simulink model "drone_estimator_angle_dynamics"  (R2024a)
settings: Solver=FixedStepAuto  StartTime=0.0  StopTime=30  FixedStep=0.001  RelTol=1e-3
InitFcn:
  | os = 0.15;
  | zeta = -log(os)/sqrt(pi^2+(log(os))^2);
  | ts = 0.2;
  | wn = 4/zeta/ts;
  | kx = wn^2 - 1;
  | kf = 2 * zeta * wn;
  | Kx = eye(2) * kx;
  | Kf = eye(2) * kf;
  | 
  | 
  | os_des = 0.1;
  | zeta_des = -log(os_des)/sqrt(pi^2+(log(os_des))^2);
  | ts_des = 1;
  | wn_des = 4/zeta_des/ts_des;
  | b_des = wn_des^2;
  | a_des = 2 * zeta_des * wn_des;
undefined symbols (not defined in the file or in its folder): e0_0, e1_0, e2_0, e3_0, q0, QP, vec
libraries: sharedtransform x12, dspsigops x12, sharedutil x6, simulink x3
(part 2 of 2)

== system drone_estimator_angle_dynamics/Quaternion Command/Filtering Command Signal ==
  Command : Inport
  In Bus Element : Inport  Port=2  PortName=States  Element=Euler.ϕ
  In Bus Element2 : Inport  Port=2  PortName=States  Element=Euler.θ
  In Bus Element1 : Inport  Port=2  PortName=States  Element=Euler.Ψ
  Demux : Demux  Outputs=3
  Mux : Mux  Inputs=3
  Pitch Dynamic Sat : Subsystem  mask{Range=PitchRange}
      mask prompts: Range "Saturation Range"
      mask TypeOptions Range: range/Value
  Pitch Rate Limiter : RateLimiter  RisingSlewLimit=PitchRisingSlewLimit  FallingSlewLimit=PitchFallingSlewLimit  SampleTimeMode=inherited
  Roll Dynamic Sat : Subsystem  mask{Range=RollRange}
      mask prompts: Range "Saturation Range"
      mask TypeOptions Range: range/Value
  Roll Rate Limiter : RateLimiter  RisingSlewLimit=RollRisingSlewLimit  FallingSlewLimit=RollFallingSlewLimit  SampleTimeMode=inherited
  Yaw Dynamic Sat : Subsystem  mask{Range=YawRange}
      mask prompts: Range "Saturation Range"
      mask TypeOptions Range: range/Value
  Yaw Rate Limiter : RateLimiter  RisingSlewLimit=YawRisingSlewLimit  FallingSlewLimit=YawFallingSlewLimit  SampleTimeMode=inherited
  Filtered : Outport
  wires:
  Yaw Dynamic Sat/1(Saturated Command) -> Yaw Rate Limiter/1
  Mux/1 -> Filtered/1
  Pitch Dynamic Sat/1(Saturated Command) -> Pitch Rate Limiter/1
  Demux/3 -> Yaw Dynamic Sat/2(Command)
  Demux/1 -> Roll Dynamic Sat/2(Command)
  In Bus Element/1 -> Roll Dynamic Sat/1(State)
  Roll Dynamic Sat/1(Saturated Command) -> Roll Rate Limiter/1
  Demux/2 -> Pitch Dynamic Sat/2(Command)
  Command/1 -> Demux/1
  In Bus Element1/1 -> Yaw Dynamic Sat/1(State)
  In Bus Element2/1 -> Pitch Dynamic Sat/1(State)
  Roll Rate Limiter/1 -> Mux/1
  Pitch Rate Limiter/1 -> Mux/2
  Yaw Rate Limiter/1 -> Mux/3

== system drone_estimator_angle_dynamics/Quaternion Command/Rotation Interpolation ==
  DCM : Inport
  In Bus Element1 : Inport  Port=2  PortName=States  Element=Quat
  In Bus Element : Inport  Port=2  PortName=States  Element=Euler
  Quaternion Interpolation : QuatInterp
  Quaternions to Direction Cosine Matrix1 : sharedtransform/Quaternions to  Direction Cosine Matrix  aMode=aMode
      settings: LibrarySourceBlock=|
      | aerolibtransform2/Quaternions to
      | Direction Cosine Matrix
  Subsystem : Subsystem
  Sum1 : Sum  Inputs=|+-
  alpha : Subsystem
  Rot : Outport
  wires:
  Subsystem/2(angles) -> Sum1/1
  Quaternion Interpolation/1 -> Quaternions to Direction Cosine Matrix1/1
  Quaternions to Direction Cosine Matrix1/1 -> Rot/1
  alpha/1(alpha) -> Quaternion Interpolation/3
  In Bus Element1/1 -> Quaternion Interpolation/1
  Subsystem/1(Quaternion) -> Quaternion Interpolation/2
  Sum1/1 -> alpha/1(angle difference)
  DCM/1 -> Subsystem/1(DCM)
  In Bus Element/1 -> Sum1/2

== system drone_estimator_angle_dynamics/Quaternion Command/ToGo ==
  DCM : Inport
  Bus Creator3 : BusCreator  Inputs=3
  Demux3 : Demux  Outputs=3
  Direction Cosine Matrix to Rotation Angles : sharedtransform/Direction Cosine Matrix to Rotation Angles  rotationOrder=ZYX  aMode=aMode  action=None  tolerance=eps(2)
      settings: LibrarySourceBlock=|
      | aerolibtransform2/Direction Cosine Matrix
      | to Rotation Angles
  Selector1 : Selector  InputPortWidth=3  IndexOptions=Index vector (dialog)  Indices=[3 2 1]  OutputSizes=1
  Unwrap2 : dspsigops/Unwrap  tol=2*pi  InputProcessing=Columns as channels (frame based)  running=off
  Unwrap3 : dspsigops/Unwrap  tol=2*pi  InputProcessing=Columns as channels (frame based)  running=off
  Unwrap4 : dspsigops/Unwrap  tol=2*pi  InputProcessing=Columns as channels (frame based)  running=off
  tag scope: Euler_c=global
  wires:
  Unwrap3/1 -> Bus Creator3/1  "ϕc"
  Demux3/1 -> Unwrap3/1
  Unwrap2/1 -> Bus Creator3/2  "θc"
  Demux3/3 -> Unwrap4/1  "Ψc"
  Bus Creator3/1 -> [Euler_c]
  Direction Cosine Matrix to Rotation Angles/1 -> Selector1/1
  Demux3/2 -> Unwrap2/1
  DCM/1 -> Demux3/1
  Unwrap4/1 -> Bus Creator3/3  "Ψc"

== system drone_estimator_angle_dynamics/Quaternion Command/quaternion ==
  angle : Inport
  vec : Inport  Port=2
  Gain : Gain  Gain=1/2
  Mux : Mux  Inputs=2
  Product : Product
  Quaternion Normalize : sharedutil/Quaternion Normalize  aMode=aMode
  Quaternions to Direction Cosine Matrix : sharedtransform/Quaternions to  Direction Cosine Matrix  aMode=aMode
      settings: LibrarySourceBlock=|
      | aerolibtransform2/Quaternions to
      | Direction Cosine Matrix
  Rate Limiter : RateLimiter  RisingSlewLimit=0.4  FallingSlewLimit=-0.4  SampleTimeMode=inherited
  Trigonometric Function : Trigonometry
  Trigonometric Function1 : Trigonometry  Operator=cos
  rot : Outport
  wires:
  Trigonometric Function1/1 -> Mux/1
  Mux/1 -> Quaternion Normalize/1
  Product/1 -> Mux/2
  Trigonometric Function/1 -> Product/1
  Gain/1 -> Trigonometric Function1/1, Trigonometric Function/1
  Rate Limiter/1 -> Product/2
  angle/1 -> Gain/1
  Quaternion Normalize/1 -> Quaternions to Direction Cosine Matrix/1
  vec/1 -> Rate Limiter/1
  Quaternions to Direction Cosine Matrix/1 -> rot/1

== system drone_estimator_angle_dynamics/Quaternion Command/to Rotation Mat ==
  Euler : Inport
  Rotation Angles to Direction Cosine Matrix : sharedtransform/Rotation Angles to Direction Cosine Matrix  rotationOrder=ZYX  aMode=aMode
  Selector : Selector  InputPortWidth=3  IndexOptions=Index vector (dialog)  Indices=[3 2 1]  OutputSizes=1
  rot : Outport
  wires:
  Selector/1 -> Rotation Angles to Direction Cosine Matrix/1
  Rotation Angles to Direction Cosine Matrix/1 -> rot/1
  Euler/1 -> Selector/1

== system drone_estimator_angle_dynamics/Rotational Matrix Controller/Quaternion Dynamics ==
  R : Inport
  Add2 : Sum  Inputs=|+-
  "Desired Rotaion Dynamic Gain " : Gain  Gain=DesiredRotaionDynamciGain
  Euler Command : Subsystem
  Euler Desired : Subsystem
  Quaternion Command : Subsystem
  Rotaion Integration : Integrator  InitialCondition=InitialCondition  ContinuousStateAttributes='qd'
  Scope : Scope
  Rd : Outport
  Rd_dot : Outport  Port=2
  wires:
  Rotaion Integration/1 -> Euler Desired/1(DCM), Add2/2, Rd/1, Scope/1
  Add2/1 -> Rd_dot/1, "Desired Rotaion Dynamic Gain "/1
  "Desired Rotaion Dynamic Gain "/1 -> Rotaion Integration/1
  R/1 -> Quaternion Command/1(DCM), Euler Command/1(DCM), Add2/1

== system drone_estimator_angle_dynamics/Rotational Matrix Controller/Rotational Controller ==
  Rd : Inport
  Rd_dot : Inport  Port=2
  Rot : Inport  Port=3
  Kr : Constant  Value=RotationControlGain
  MATLAB Function : MATLAB Function  TreatAsAtomicUnit=on
  MATLAB Function1 : MATLAB Function  TreatAsAtomicUnit=on
  Manual Switch : ManualSwitch  CurrentSetting=0
  Manual Switch2 : ManualSwitch  CurrentSetting=0
  "Rd " : InportShadow
  "Rd_dot " : InportShadow  Port=2
  "Rot " : InportShadow  Port=3
  Scope : Scope
  Scope1 : Scope
  wc : Outport
  tag scope: sr=global
  wires:
  Rd/1 -> MATLAB Function/3(Rd)
  MATLAB Function/1(sr) -> Manual Switch2/1
  Kr/1 -> MATLAB Function1/1(Kr), MATLAB Function/1(Kr)
  MATLAB Function/2(wc) -> Manual Switch/1
  Rd_dot/1 -> MATLAB Function/4(Rd_dot)
  Manual Switch/1 -> wc/1
  "Rd_dot "/1 -> MATLAB Function1/4(Rd_dot)
  "Rd "/1 -> MATLAB Function1/3(Rd)
  MATLAB Function1/2(wc) -> Manual Switch/2
  MATLAB Function/3(Re) -> Scope/1
  Manual Switch2/1 -> [sr]
  MATLAB Function1/1(sr) -> Manual Switch2/2
  MATLAB Function1/3(Re) -> Scope1/1
  "Rot "/1 -> MATLAB Function1/2(R)
  Rot/1 -> MATLAB Function/2(R)

== system drone_estimator_angle_dynamics/Angular Rate Controller/Dynamic Surface Angular Rate Controller/Angular Rate Desired Dynamics ==
  wc : Inport
  Desired Angular Rate Integaration : Integrator  InitialCondition=DesiredAngularRateInitCond
  Sum : Sum  Inputs=|+-
  tau : Gain  Gain=OmegaTimeConstant
  wd : Outport
  wd dot : Outport  Port=2
  wires:
  Sum/1 -> tau/1
  Desired Angular Rate Integaration/1 -> wd/1, Sum/2
  wc/1 -> Sum/1
  tau/1 -> wd dot/1, Desired Angular Rate Integaration/1

== system drone_estimator_angle_dynamics/Estimator/Model Predictor/Nonlinear function estimator ==
  e : Inport
  Add1 : Sum
  Gain : Gain  Gain=5
  Gain1 : Gain  Gain=2
  Integrator : Integrator
  fest : Outport
  tag scope: Fest=global
  wires:
  e/1 -> Gain1/1, Integrator/1
  Gain1/1 -> Add1/1
  Add1/1 -> fest/1, [Fest]
  Gain/1 -> Add1/2
  Integrator/1 -> Gain/1

== system drone_estimator_angle_dynamics/Estimator/Model Predictor/Subsystem1 ==
  xe : Inport
  x : Inport  Port=2
  Bus Creator1 : BusCreator  Inputs=3
  Bus Selector : BusSelector  OutputSignals=w.p,w.q,w.r  OutputAsBus=on
  Bus Selector1 : BusSelector  OutputSignals=p,q,r  OutputAsBus=on
  Demux : Demux  Outputs=3
  Reshape1 : Reshape  OutputDimensionality=Column vector (2-D)
  Reshape4 : Reshape  OutputDimensionality=Column vector (2-D)
  Subtract : Sum  Inputs=+-
  er : Outport
  tag scope: we_est=global
  wires:
  Demux/3 -> Bus Creator1/3  "er"
  Reshape4/1 -> Subtract/1
  Bus Selector1/1 -> Reshape1/1
  Reshape1/1 -> Subtract/2
  Demux/2 -> Bus Creator1/2  "eq"
  x/1 -> Bus Selector/1
  Bus Creator1/1 -> [we_est]
  Demux/1 -> Bus Creator1/1  "ep"
  Bus Selector/1 -> Reshape4/1
  xe/1 -> Bus Selector1/1
  Subtract/1 -> Demux/1, er/1

== system drone_estimator_angle_dynamics/Estimator/Model Predictor1/Centrifugal Moments ==
  ω : Inport
  Inertia : Inport  Port=2
  3x3 Cross Product : sharedutil/3x3 Cross Product  aMode=aMode
  Product : Product  Multiplication=Matrix(*)  InputSameDT=on  SaturateOnIntegerOverflow=on  OutDataTypeStr=Inherit: Same as first input
  To1D : Reshape
  ToVec : Reshape  OutputDimensionality=Column vector (2-D)
  (I * ω) x ω : Outport
  wires:
  Inertia/1 -> Product/1
  To1D/1 -> 3x3 Cross Product/1  "I * ω"
  3x3 Cross Product/1 -> (I * ω) x ω/1
  ω/1 -> ToVec/1, 3x3 Cross Product/2
  Product/1 -> To1D/1
  ToVec/1 -> Product/2

== system drone_estimator_angle_dynamics/Estimator/Model Predictor1/Subsystem ==
  (I * ω) x ω : Inport
  e : Inport  Port=2
  Add1 : Sum  Inputs=+++
  Gain : Gain  Gain=5
  Gain1 : Gain  Gain=2
  Integrator : Integrator
  fest : Outport
  tag scope: Fest=global
  wires:
  (I * ω) x ω/1 -> Add1/3
  Integrator/1 -> Gain/1
  Gain/1 -> Add1/2
  Add1/1 -> [Fest], fest/1
  Gain1/1 -> Add1/1
  e/1 -> Integrator/1, Gain1/1

== system drone_estimator_angle_dynamics/Estimator/Model Predictor1/Subsystem1 ==
  xe : Inport
  x : Inport  Port=2
  Bus Creator1 : BusCreator  Inputs=3
  Bus Selector : BusSelector  OutputSignals=w.p,w.q,w.r  OutputAsBus=on
  Bus Selector1 : BusSelector  OutputSignals=p,q,r  OutputAsBus=on
  Demux : Demux  Outputs=3
  Reshape1 : Reshape  OutputDimensionality=Column vector (2-D)
  Reshape4 : Reshape  OutputDimensionality=Column vector (2-D)
  Subtract : Sum  Inputs=+-
  er : Outport
  tag scope: we_est=global
  wires:
  Subtract/1 -> Demux/1
  xe/1 -> Bus Selector1/1
  Bus Selector/1 -> Reshape4/1
  Demux/1 -> Bus Creator1/1  "ep"
  Bus Creator1/1 -> er/1, [we_est]
  x/1 -> Bus Selector/1
  Demux/2 -> Bus Creator1/2  "eq"
  Reshape1/1 -> Subtract/2
  Bus Selector1/1 -> Reshape1/1
  Reshape4/1 -> Subtract/1
  Demux/3 -> Bus Creator1/3  "er"

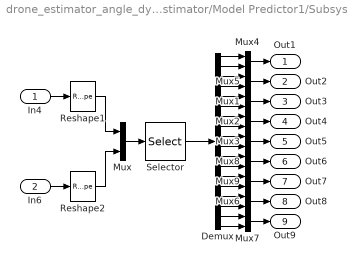
== system drone_estimator_angle_dynamics/Estimator/Model Predictor1/Subsystem2 ==
  In4 : Inport
  In6 : Inport  Port=2
  Demux : Demux  Outputs=18
  Mux{,1..9} (10 alike) : Mux  Inputs=2
  Reshape1 : Reshape
  Reshape2 : Reshape
  Selector : Selector  InputPortWidth=18  IndexOptions=Index vector (dialog)  Indices=[1 10 2 11 3 12 4 13 5 14 6 15 7 16 8 17 9 18]  OutputSizes=1
  Out1 : Outport
  Out2 : Outport  Port=2
  Out3 : Outport  Port=3
  Out4 : Outport  Port=4
  Out5 : Outport  Port=5
  Out6 : Outport  Port=6
  Out7 : Outport  Port=7
  Out8 : Outport  Port=8
  Out9 : Outport  Port=9
  wires:
  Demux/12 -> Mux8/2
  Demux/13 -> Mux9/1
  Demux/14 -> Mux9/2
  Demux/15 -> Mux6/1
  Demux/16 -> Mux6/2
  Demux/17 -> Mux7/1
  Demux/18 -> Mux7/2
  Demux/11 -> Mux8/1
  Demux/10 -> Mux3/2
  Demux/9 -> Mux3/1
  Demux/8 -> Mux2/2
  Demux/7 -> Mux2/1
  Demux/6 -> Mux1/2
  Demux/5 -> Mux1/1
  Demux/4 -> Mux5/2
  Demux/3 -> Mux5/1
  Demux/2 -> Mux4/2
  Demux/1 -> Mux4/1
  Selector/1 -> Demux/1
  Mux/1 -> Selector/1
  Mux8/1 -> Out6/1
  Mux9/1 -> Out7/1
  Mux7/1 -> Out9/1
  Mux6/1 -> Out8/1
  Mux3/1 -> Out5/1
  Mux1/1 -> Out3/1
  Mux2/1 -> Out4/1
  Mux5/1 -> Out2/1
  In6/1 -> Reshape2/1
  Reshape2/1 -> Mux/2
  In4/1 -> Reshape1/1
  Reshape1/1 -> Mux/1
  Mux4/1 -> Out1/1

== system drone_estimator_angle_dynamics/Estimator/Model Predictor1/Subsystem3 ==
  In1 : Inport
  In2 : Inport  Port=2
  Demux : Demux  Outputs=3
  Demux1 : Demux  Outputs=3
  Mux10 : Mux  Inputs=2
  Mux11 : Mux  Inputs=2
  Mux9 : Mux  Inputs=2
  Out1 : Outport
  Out2 : Outport  Port=2
  Out3 : Outport  Port=3
  wires:
  Demux/3 -> Mux11/1
  Mux9/1 -> Out1/1
  Demux1/1 -> Mux9/2
  Demux/2 -> Mux10/1
  Demux/1 -> Mux9/1
  Demux1/3 -> Mux11/2
  Demux1/2 -> Mux10/2
  Mux11/1 -> Out3/1
  Mux10/1 -> Out2/1
  In1/1 -> Demux/1
  In2/1 -> Demux1/1

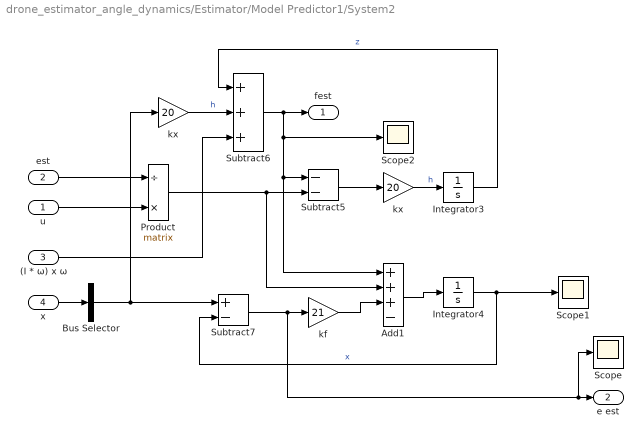
== system drone_estimator_angle_dynamics/Estimator/Model Predictor1/System2 ==
  u : Inport
  est : Inport  Port=2
  (I * ω) x ω : Inport  Port=3
  x : Inport  Port=4
  Add1 : Sum  Inputs=+++-
  Bus Selector : BusSelector  OutputSignals=w.p,w.q,w.r  OutputAsBus=on
  Integrator3 : Integrator  InitialCondition=zeros(3,1)
  Integrator4 : Integrator  InitialCondition=zeros(3,1)
  Product : Product  Inputs=/*  Multiplication=Matrix(*)
  Scope : Scope
  Scope1 : Scope
  Scope2 : Scope
  Subtract5 : Sum  Inputs=--
  Subtract6 : Sum  Inputs=+++
  Subtract7 : Sum  Inputs=+-
  kf : Gain  Gain=21
  kx : Gain  Gain=20
  "kx " : Gain  Gain=20
  fest : Outport
  e est : Outport  Port=2
  wires:
  (I * ω) x ω/1 -> Subtract6/3
  Bus Selector/1 -> kx/1, Subtract7/1
  u/1 -> Product/2
  est/1 -> Product/1
  Subtract7/1 -> kf/1, Scope/1, e est/1
  x/1 -> Bus Selector/1
  kf/1 -> Add1/3
  Integrator4/1 -> Subtract7/2, Scope1/1  "x"
  Add1/1 -> Integrator4/1
  Product/1 -> Subtract5/2, Add1/2
  Subtract6/1 -> fest/1, Subtract5/1, Add1/1, Scope2/1
  "kx "/1 -> Integrator3/1  "h"
  Subtract5/1 -> "kx "/1
  Integrator3/1 -> Subtract6/1  "z"
  kx/1 -> Subtract6/2  "h"

== system drone_estimator_angle_dynamics/Estimator1/Model Predictor/Nonlinear function estimator ==
  e : Inport
  Add1 : Sum
  Gain : Gain  Gain=5
  Gain1 : Gain  Gain=2
  Integrator : Integrator
  fest : Outport
  tag scope: Fest=global
  wires:
  Integrator/1 -> Gain/1
  Gain/1 -> Add1/2
  Add1/1 -> [Fest], fest/1
  Gain1/1 -> Add1/1
  e/1 -> Integrator/1, Gain1/1

== system drone_estimator_angle_dynamics/Estimator1/Model Predictor/Subsystem1 ==
  xe : Inport
  x : Inport  Port=2
  Bus Creator1 : BusCreator  Inputs=3
  Bus Selector : BusSelector  OutputSignals=w.p,w.q,w.r  OutputAsBus=on
  Bus Selector1 : BusSelector  OutputSignals=p,q,r  OutputAsBus=on
  Demux : Demux  Outputs=3
  Reshape1 : Reshape  OutputDimensionality=Column vector (2-D)
  Reshape4 : Reshape  OutputDimensionality=Column vector (2-D)
  Subtract : Sum  Inputs=+-
  er : Outport
  tag scope: we_est=global
  wires:
  Subtract/1 -> er/1, Demux/1
  xe/1 -> Bus Selector1/1
  Bus Selector/1 -> Reshape4/1
  Demux/1 -> Bus Creator1/1  "ep"
  Bus Creator1/1 -> [we_est]
  x/1 -> Bus Selector/1
  Demux/2 -> Bus Creator1/2  "eq"
  Reshape1/1 -> Subtract/2
  Bus Selector1/1 -> Reshape1/1
  Reshape4/1 -> Subtract/1
  Demux/3 -> Bus Creator1/3  "er"

== system drone_estimator_angle_dynamics/Estimator1/Model Predictor1/Centrifugal Moments ==
  ω : Inport
  Inertia : Inport  Port=2
  3x3 Cross Product : sharedutil/3x3 Cross Product  aMode=aMode
  Product : Product  Multiplication=Matrix(*)  InputSameDT=on  SaturateOnIntegerOverflow=on  OutDataTypeStr=Inherit: Same as first input
  To1D : Reshape
  ToVec : Reshape  OutputDimensionality=Column vector (2-D)
  (I * ω) x ω : Outport
  wires:
  ToVec/1 -> Product/2
  Product/1 -> To1D/1
  ω/1 -> 3x3 Cross Product/2, ToVec/1
  3x3 Cross Product/1 -> (I * ω) x ω/1
  To1D/1 -> 3x3 Cross Product/1  "I * ω"
  Inertia/1 -> Product/1

== system drone_estimator_angle_dynamics/Estimator1/Model Predictor1/Subsystem ==
  (I * ω) x ω : Inport
  e : Inport  Port=2
  Add1 : Sum  Inputs=+++
  Gain : Gain  Gain=5
  Gain1 : Gain  Gain=2
  Integrator : Integrator
  fest : Outport
  tag scope: Fest=global
  wires:
  e/1 -> Gain1/1, Integrator/1
  Gain1/1 -> Add1/1
  Add1/1 -> fest/1, [Fest]
  Gain/1 -> Add1/2
  Integrator/1 -> Gain/1
  (I * ω) x ω/1 -> Add1/3

== system drone_estimator_angle_dynamics/Estimator1/Model Predictor1/Subsystem1 ==
  xe : Inport
  x : Inport  Port=2
  Bus Creator1 : BusCreator  Inputs=3
  Bus Selector : BusSelector  OutputSignals=w.p,w.q,w.r  OutputAsBus=on
  Bus Selector1 : BusSelector  OutputSignals=p,q,r  OutputAsBus=on
  Demux : Demux  Outputs=3
  Reshape1 : Reshape  OutputDimensionality=Column vector (2-D)
  Reshape4 : Reshape  OutputDimensionality=Column vector (2-D)
  Subtract : Sum  Inputs=+-
  er : Outport
  tag scope: we_est=global
  wires:
  Demux/3 -> Bus Creator1/3  "er"
  Reshape4/1 -> Subtract/1
  Bus Selector1/1 -> Reshape1/1
  Reshape1/1 -> Subtract/2
  Demux/2 -> Bus Creator1/2  "eq"
  x/1 -> Bus Selector/1
  Bus Creator1/1 -> [we_est], er/1
  Demux/1 -> Bus Creator1/1  "ep"
  Bus Selector/1 -> Reshape4/1
  xe/1 -> Bus Selector1/1
  Subtract/1 -> Demux/1

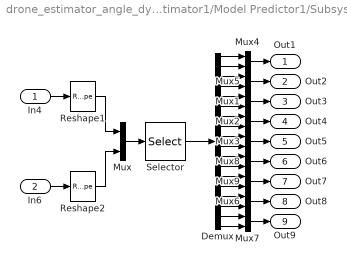
== system drone_estimator_angle_dynamics/Estimator1/Model Predictor1/Subsystem2 ==
  In4 : Inport
  In6 : Inport  Port=2
  Demux : Demux  Outputs=18
  Mux{,1..9} (10 alike) : Mux  Inputs=2
  Reshape1 : Reshape
  Reshape2 : Reshape
  Selector : Selector  InputPortWidth=18  IndexOptions=Index vector (dialog)  Indices=[1 10 2 11 3 12 4 13 5 14 6 15 7 16 8 17 9 18]  OutputSizes=1
  Out1 : Outport
  Out2 : Outport  Port=2
  Out3 : Outport  Port=3
  Out4 : Outport  Port=4
  Out5 : Outport  Port=5
  Out6 : Outport  Port=6
  Out7 : Outport  Port=7
  Out8 : Outport  Port=8
  Out9 : Outport  Port=9
  wires:
  Mux4/1 -> Out1/1
  Reshape1/1 -> Mux/1
  In4/1 -> Reshape1/1
  Reshape2/1 -> Mux/2
  In6/1 -> Reshape2/1
  Mux5/1 -> Out2/1
  Mux2/1 -> Out4/1
  Mux1/1 -> Out3/1
  Mux3/1 -> Out5/1
  Mux6/1 -> Out8/1
  Mux7/1 -> Out9/1
  Mux9/1 -> Out7/1
  Mux8/1 -> Out6/1
  Mux/1 -> Selector/1
  Selector/1 -> Demux/1
  Demux/1 -> Mux4/1
  Demux/2 -> Mux4/2
  Demux/3 -> Mux5/1
  Demux/4 -> Mux5/2
  Demux/5 -> Mux1/1
  Demux/6 -> Mux1/2
  Demux/7 -> Mux2/1
  Demux/8 -> Mux2/2
  Demux/9 -> Mux3/1
  Demux/10 -> Mux3/2
  Demux/11 -> Mux8/1
  Demux/18 -> Mux7/2
  Demux/17 -> Mux7/1
  Demux/16 -> Mux6/2
  Demux/15 -> Mux6/1
  Demux/14 -> Mux9/2
  Demux/13 -> Mux9/1
  Demux/12 -> Mux8/2

== system drone_estimator_angle_dynamics/Estimator1/Model Predictor1/Subsystem3 ==
  In1 : Inport
  In2 : Inport  Port=2
  Demux : Demux  Outputs=3
  Demux1 : Demux  Outputs=3
  Mux10 : Mux  Inputs=2
  Mux11 : Mux  Inputs=2
  Mux9 : Mux  Inputs=2
  Out1 : Outport
  Out2 : Outport  Port=2
  Out3 : Outport  Port=3
  wires:
  In2/1 -> Demux1/1
  In1/1 -> Demux/1
  Mux10/1 -> Out2/1
  Mux11/1 -> Out3/1
  Demux1/2 -> Mux10/2
  Demux1/3 -> Mux11/2
  Demux/1 -> Mux9/1
  Demux/2 -> Mux10/1
  Demux1/1 -> Mux9/2
  Mux9/1 -> Out1/1
  Demux/3 -> Mux11/1

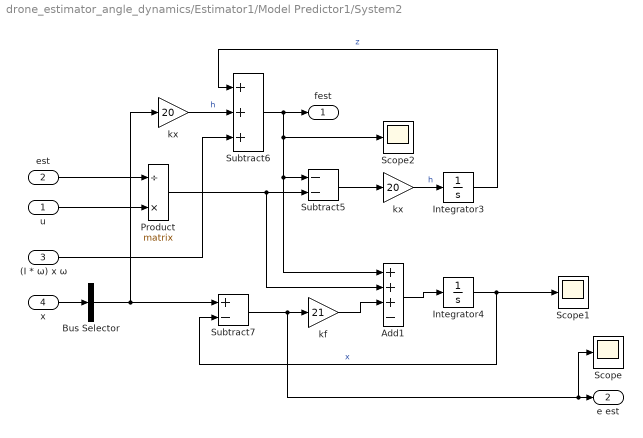
== system drone_estimator_angle_dynamics/Estimator1/Model Predictor1/System2 ==
  u : Inport
  est : Inport  Port=2
  (I * ω) x ω : Inport  Port=3
  x : Inport  Port=4
  Add1 : Sum  Inputs=+++-
  Bus Selector : BusSelector  OutputSignals=w.p,w.q,w.r  OutputAsBus=on
  Integrator3 : Integrator  InitialCondition=zeros(3,1)
  Integrator4 : Integrator  InitialCondition=zeros(3,1)
  Product : Product  Inputs=/*  Multiplication=Matrix(*)
  Scope : Scope
  Scope1 : Scope
  Scope2 : Scope
  Subtract5 : Sum  Inputs=--
  Subtract6 : Sum  Inputs=+++
  Subtract7 : Sum  Inputs=+-
  kf : Gain  Gain=21
  kx : Gain  Gain=20
  "kx " : Gain  Gain=20
  fest : Outport
  e est : Outport  Port=2
  wires:
  kx/1 -> Subtract6/2  "h"
  Integrator3/1 -> Subtract6/1  "z"
  Subtract5/1 -> "kx "/1
  "kx "/1 -> Integrator3/1  "h"
  Subtract6/1 -> Scope2/1, Add1/1, Subtract5/1, fest/1
  Product/1 -> Add1/2, Subtract5/2
  Add1/1 -> Integrator4/1
  Integrator4/1 -> Scope1/1, Subtract7/2  "x"
  kf/1 -> Add1/3
  x/1 -> Bus Selector/1
  Subtract7/1 -> e est/1, Scope/1, kf/1
  est/1 -> Product/1
  u/1 -> Product/2
  Bus Selector/1 -> Subtract7/1, kx/1
  (I * ω) x ω/1 -> Subtract6/3

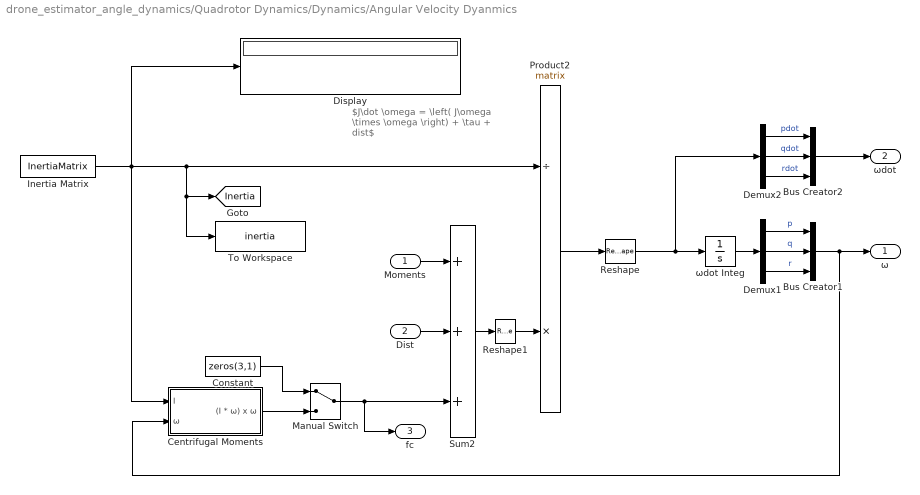
== system drone_estimator_angle_dynamics/Quadrotor Dynamics/Dynamics/Angular Velocity Dyanmics ==
  note: $J\dot \omega = \left( J\omega \times \omega \right) + \tau + dist$
  Moments : Inport  OutDataTypeStr=double
  Dist : Inport  Port=2  OutDataTypeStr=double
  Bus Creator1 : BusCreator  Inputs=3
  Bus Creator2 : BusCreator  Inputs=3
  Centrifugal Moments : Subsystem
  Constant : Constant  Value=zeros(3,1)
  Demux1 : Demux  Outputs=3
  Demux2 : Demux  Outputs=3
  Display : Display
  Inertia Matrix : Constant  Value=InertiaMatrix
  Manual Switch : ManualSwitch
  Product2 : Product  Inputs=/*  Multiplication=Matrix(*)  SaturateOnIntegerOverflow=on  OutDataTypeStr=Inherit: Same as first input
  Reshape : Reshape
  Reshape1 : Reshape  OutputDimensionality=Column vector (2-D)
  Sum2 : Sum  Inputs=+++  SaturateOnIntegerOverflow=on
  To Workspace : ToWorkspace  VariableName=inertia  SampleTime=-1
      settings: Save2DSignal=2-D array (concatenate along first dimension)
  ωdot Integ : Integrator  InitialCondition=OmegaInitialValues  ContinuousStateAttributes={'p', 'q', 'r'}
  ω : Outport
  ωdot : Outport  Port=2  OutDataTypeStr=double  Unit=rad/s^2  VectorParamsAs1DForOutWhenUnconnected=off
  fc : Outport  Port=3
  tag scope: Inertia=global
  wires:
  Product2/1 -> Reshape/1
  Reshape1/1 -> Product2/2
  Demux1/1 -> Bus Creator1/1  "p"
  ωdot Integ/1 -> Demux1/1
  Demux1/3 -> Bus Creator1/3  "r"
  Demux1/2 -> Bus Creator1/2  "q"
  Bus Creator1/1 -> ω/1, Centrifugal Moments/2(ω)
  Sum2/1 -> Reshape1/1
  Reshape/1 -> ωdot Integ/1, Demux2/1
  Demux2/2 -> Bus Creator2/2  "qdot"
  Demux2/3 -> Bus Creator2/3  "rdot"
  Demux2/1 -> Bus Creator2/1  "pdot"
  Bus Creator2/1 -> ωdot/1
  Inertia Matrix/1 -> To Workspace/1, [Inertia], Product2/1, Display/1, Centrifugal Moments/1(I)
  Moments/1 -> Sum2/1
  Manual Switch/1 -> fc/1, Sum2/3
  Centrifugal Moments/1((I * ω) x ω) -> Manual Switch/2
  Constant/1 -> Manual Switch/1
  Dist/1 -> Sum2/2

== system drone_estimator_angle_dynamics/Quadrotor Dynamics/Dynamics/Mixer ==
  Omegas : Inport
  Bus Creator : BusCreator  Inputs=4
  Constant : Constant  Value=ThustForceCoefficient
  Demux : Demux
  Matrix Multiply : Product  Multiplication=Matrix(*)
  Square : Math  Operator=square
  U : Outport
  wires:
  Bus Creator/1 -> U/1
  Demux/4 -> Bus Creator/4  "Tz"
  Demux/3 -> Bus Creator/3  "Ty"
  Demux/2 -> Bus Creator/2  "Tx"
  Demux/1 -> Bus Creator/1  "Th"
  Constant/1 -> Matrix Multiply/1
  Matrix Multiply/1 -> Demux/1
  Omegas/1 -> Matrix Multiply/2

== system drone_estimator_angle_dynamics/Quadrotor Dynamics/Dynamics/Quaternion Dynamics ==
  ω : Inport
  Quat to Euler : Subsystem
  Quaternion Dynamics : Subsystem
  Rotational Dynamics : Subsystem
  DCM_be : Outport  OutDataTypeStr=double  VectorParamsAs1DForOutWhenUnconnected=off
  Quat : Outport  Port=2  OutDataTypeStr=double  VectorParamsAs1DForOutWhenUnconnected=off
  Euler : Outport  Port=3  OutDataTypeStr=double  VectorParamsAs1DForOutWhenUnconnected=off
  wires:
  Quaternion Dynamics/1(qdot) -> Quat/1
  Rotational Dynamics/1(Rbe) -> Quat to Euler/1(Rot), DCM_be/1
  Quat to Euler/1(euler) -> Euler/1
  ω/1 -> Rotational Dynamics/1(w), Quaternion Dynamics/1(ω)

== system drone_estimator_angle_dynamics/Quaternion Command/Filtering Command Signal/Pitch Dynamic Sat ==
  State : Inport
  Command : Inport  Port=2
  Add : Sum
  Add1 : Sum
  Saturation Dynamic : simulink/Discontinuities/Saturation Dynamic  OutMin=[]  OutMax=[]  OutDataTypeStr=Inherit: Same as second input  OutDataType=fixdt(1, 16)  OutScaling=2^-10  DoSatur=off
  Unary Minus : UnaryMinus
  range : Constant  Value=Range
  Saturated Command : Outport
  wires:
  Add1/1 -> Saturation Dynamic/3
  Saturation Dynamic/1 -> Saturated Command/1
  range/1 -> Unary Minus/1, Add/1
  State/1 -> Add/2, Add1/1
  Add/1 -> Saturation Dynamic/1
  Unary Minus/1 -> Add1/2
  Command/1 -> Saturation Dynamic/2

== system drone_estimator_angle_dynamics/Quaternion Command/Filtering Command Signal/Roll Dynamic Sat ==
  State : Inport
  Command : Inport  Port=2
  Add : Sum
  Add1 : Sum
  Saturation Dynamic : simulink/Discontinuities/Saturation Dynamic  OutMin=[]  OutMax=[]  OutDataTypeStr=Inherit: Same as second input  OutDataType=fixdt(1, 16)  OutScaling=2^-10  DoSatur=off
  Unary Minus : UnaryMinus
  range : Constant  Value=Range
  Saturated Command : Outport
  wires:
  Command/1 -> Saturation Dynamic/2
  Unary Minus/1 -> Add1/2
  Add/1 -> Saturation Dynamic/1
  State/1 -> Add1/1, Add/2
  range/1 -> Add/1, Unary Minus/1
  Saturation Dynamic/1 -> Saturated Command/1
  Add1/1 -> Saturation Dynamic/3

== system drone_estimator_angle_dynamics/Quaternion Command/Filtering Command Signal/Yaw Dynamic Sat ==
  State : Inport
  Command : Inport  Port=2
  Add : Sum
  Add1 : Sum
  Saturation Dynamic : simulink/Discontinuities/Saturation Dynamic  OutMin=[]  OutMax=[]  OutDataTypeStr=Inherit: Same as second input  OutDataType=fixdt(1, 16)  OutScaling=2^-10  DoSatur=off
  Unary Minus : UnaryMinus
  range : Constant  Value=Range
  Saturated Command : Outport
  wires:
  Command/1 -> Saturation Dynamic/2
  Unary Minus/1 -> Add1/2
  Add/1 -> Saturation Dynamic/1
  State/1 -> Add1/1, Add/2
  range/1 -> Add/1, Unary Minus/1
  Saturation Dynamic/1 -> Saturated Command/1
  Add1/1 -> Saturation Dynamic/3

== system drone_estimator_angle_dynamics/Quaternion Command/Rotation Interpolation/Subsystem ==
  DCM : Inport
  Direction Cosine Matrix to Rotation Angles : sharedtransform/Direction Cosine Matrix to Rotation Angles  rotationOrder=ZYX  aMode=aMode  action=None  tolerance=eps(2)
      settings: LibrarySourceBlock=|
      | aerolibtransform2/Direction Cosine Matrix
      | to Rotation Angles
  Direction Cosine Matrix to Quaternions1 : sharedtransform/Direction Cosine Matrix  to Quaternions  aMode=0  action=None  tolerance=eps(2)
      settings: LibrarySourceBlock=|
      | aerolibtransform2/Direction Cosine Matrix
      | to Quaternions
  Selector1 : Selector  InputPortWidth=3  IndexOptions=Index vector (dialog)  Indices=[3 2 1]  OutputSizes=1
  Quaternion : Outport
  angles : Outport  Port=2
  wires:
  Selector1/1 -> angles/1
  Direction Cosine Matrix to Rotation Angles/1 -> Selector1/1
  DCM/1 -> Direction Cosine Matrix to Quaternions1/1, Direction Cosine Matrix to Rotation Angles/1
  Direction Cosine Matrix to Quaternions1/1 -> Quaternion/1

== system drone_estimator_angle_dynamics/Quaternion Command/Rotation Interpolation/alpha ==
  angle difference : Inport
  Demux : Demux  Outputs=3
  Gain2 : Gain  Gain=6/5
  Guassian (a)1 : Subsystem
  Guassian (a)2 : Subsystem
  Guassian (a)3 : Subsystem
  Saturation : Saturate  UpperLimit=1  LowerLimit=0
  Sum2 : Sum  Inputs=+++
  alpha : Outport
  wires:
  Demux/1 -> Guassian (a)1/1(In1)
  Sum2/1 -> Gain2/1
  Demux/3 -> Guassian (a)3/1(In1)
  Demux/2 -> Guassian (a)2/1(In1)
  angle difference/1 -> Demux/1
  Gain2/1 -> Saturation/1
  Saturation/1 -> alpha/1
  Guassian (a)1/1(Out1) -> Sum2/1
  Guassian (a)3/1(Out1) -> Sum2/3
  Guassian (a)2/1(Out1) -> Sum2/2

== system drone_estimator_angle_dynamics/Rotational Matrix Controller/Quaternion Dynamics/Euler Command ==
  DCM : Inport
  Bus Creator3 : BusCreator  Inputs=3
  Demux3 : Demux  Outputs=3
  Direction Cosine Matrix to Rotation Angles : sharedtransform/Direction Cosine Matrix to Rotation Angles  rotationOrder=ZYX  aMode=aMode  action=None  tolerance=eps(2)
      settings: LibrarySourceBlock=|
      | aerolibtransform2/Direction Cosine Matrix
      | to Rotation Angles
  Scope : Scope
  Selector1 : Selector  InputPortWidth=3  IndexOptions=Index vector (dialog)  Indices=[3 2 1]  OutputSizes=1
  Unwrap : dspsigops/Unwrap  tol=pi  InputProcessing=Columns as channels (frame based)  running=off
  Unwrap1 : dspsigops/Unwrap  tol=pi  InputProcessing=Columns as channels (frame based)  running=off
  Unwrap2 : dspsigops/Unwrap  tol=pi  InputProcessing=Columns as channels (frame based)  running=off
  wires:
  DCM/1 -> Direction Cosine Matrix to Rotation Angles/1
  Demux3/1 -> Unwrap2/1  "ϕc"
  Direction Cosine Matrix to Rotation Angles/1 -> Selector1/1
  Unwrap/1 -> Bus Creator3/3  "Ψc"
  Demux3/3 -> Unwrap/1
  Selector1/1 -> Demux3/1
  Demux3/2 -> Unwrap1/1  "θc"
  Unwrap1/1 -> Bus Creator3/2  "θc"
  Unwrap2/1 -> Bus Creator3/1  "ϕc"
  Bus Creator3/1 -> Scope/1

== system drone_estimator_angle_dynamics/Rotational Matrix Controller/Quaternion Dynamics/Euler Desired ==
  DCM : Inport
  Bus Creator1 : BusCreator  Inputs=3
  Demux1 : Demux  Outputs=3
  Direction Cosine Matrix to Rotation Angles : sharedtransform/Direction Cosine Matrix to Rotation Angles  rotationOrder=ZYX  aMode=aMode  action=None  tolerance=eps(2)
      settings: LibrarySourceBlock=|
      | aerolibtransform2/Direction Cosine Matrix
      | to Rotation Angles
  Selector : Selector  InputPortWidth=3  IndexOptions=Index vector (dialog)  Indices=[3 2 1]  OutputSizes=1
  Unwrap1 : dspsigops/Unwrap  tol=pi  InputProcessing=Columns as channels (frame based)  running=off
  Unwrap2 : dspsigops/Unwrap  tol=pi  InputProcessing=Columns as channels (frame based)  running=off
  Unwrap3 : dspsigops/Unwrap  tol=pi  InputProcessing=Columns as channels (frame based)  running=off
  tag scope: Euler_d=global
  wires:
  DCM/1 -> Direction Cosine Matrix to Rotation Angles/1
  Demux1/3 -> Unwrap1/1
  Demux1/1 -> Unwrap3/1
  Selector/1 -> Demux1/1
  Bus Creator1/1 -> [Euler_d]
  Unwrap1/1 -> Bus Creator1/3  "Ψd"
  Direction Cosine Matrix to Rotation Angles/1 -> Selector/1
  Demux1/2 -> Unwrap2/1
  Unwrap2/1 -> Bus Creator1/2  "θd"
  Unwrap3/1 -> Bus Creator1/1  "ϕd"

== system drone_estimator_angle_dynamics/Rotational Matrix Controller/Quaternion Dynamics/Quaternion Command ==
  DCM : Inport
  Bus Creator1 : BusCreator  Inputs=q0,vec  OutDataTypeStr=Bus: QuaturnionBus
  Demux2 : Demux
  Direction Cosine Matrix to Quaternions : sharedtransform/Direction Cosine Matrix  to Quaternions  aMode=0  action=None  tolerance=eps(2)
      settings: LibrarySourceBlock=|
      | aerolibtransform2/Direction Cosine Matrix
      | to Quaternions
  Mux : Mux  Inputs=3
  tag scope: qc=global
  wires:
  DCM/1 -> Direction Cosine Matrix to Quaternions/1
  Mux/1 -> Bus Creator1/2  "vec"
  Demux2/1 -> Bus Creator1/1  "q0"
  Demux2/2 -> Mux/1
  Demux2/3 -> Mux/2
  Demux2/4 -> Mux/3
  Direction Cosine Matrix to Quaternions/1 -> Demux2/1
  Bus Creator1/1 -> [qc]

== system drone_estimator_angle_dynamics/Quadrotor Dynamics/Dynamics/Angular Velocity Dyanmics/Centrifugal Moments ==
  I : Inport
  ω : Inport  Port=2
  3x3 Cross Product : sharedutil/3x3 Cross Product  aMode=aMode
  Product : Product  Multiplication=Matrix(*)  InputSameDT=on  SaturateOnIntegerOverflow=on  OutDataTypeStr=Inherit: Same as first input
  To1D : Reshape
  ToVec : Reshape  OutputDimensionality=Column vector (2-D)
  (I * ω) x ω : Outport
  wires:
  ToVec/1 -> Product/2
  Product/1 -> To1D/1
  I/1 -> Product/1
  ω/1 -> 3x3 Cross Product/2, ToVec/1
  3x3 Cross Product/1 -> (I * ω) x ω/1
  To1D/1 -> 3x3 Cross Product/1  "I * ω"

== system drone_estimator_angle_dynamics/Quadrotor Dynamics/Dynamics/Quaternion Dynamics/Quat to Euler ==
  Rot : Inport
  Bus Creator3 : BusCreator  Inputs=3
  Demux3 : Demux  Outputs=3
  Direction Cosine Matrix to Rotation Angles : sharedtransform/Direction Cosine Matrix to Rotation Angles  rotationOrder=ZYX  aMode=aMode  action=None  tolerance=eps(2)
      settings: LibrarySourceBlock=|
      | aerolibtransform2/Direction Cosine Matrix
      | to Rotation Angles
  Selector : Selector  InputPortWidth=3  IndexOptions=Index vector (dialog)  Indices=[3 2 1]  OutputSizes=1
  Unwrap1 : dspsigops/Unwrap  tol=2*pi  InputProcessing=Columns as channels (frame based)  running=off
  Unwrap3 : dspsigops/Unwrap  tol=2*pi  InputProcessing=Columns as channels (frame based)  running=off
  Unwrap4 : dspsigops/Unwrap  tol=2*pi  InputProcessing=Columns as channels (frame based)  running=off
  euler : Outport
  wires:
  Direction Cosine Matrix to Rotation Angles/1 -> Selector/1
  Rot/1 -> Direction Cosine Matrix to Rotation Angles/1
  Selector/1 -> Demux3/1
  Bus Creator3/1 -> euler/1
  Demux3/2 -> Unwrap1/1
  Demux3/1 -> Unwrap3/1
  Demux3/3 -> Unwrap4/1
  Unwrap1/1 -> Bus Creator3/2  "θ"
  Unwrap3/1 -> Bus Creator3/1  "ϕ"
  Unwrap4/1 -> Bus Creator3/3  "Ψ"

== system drone_estimator_angle_dynamics/Quadrotor Dynamics/Dynamics/Quaternion Dynamics/Quaternion Dynamics ==
  ω : Inport  OutDataTypeStr=double
  Integrating : Subsystem
  Quaternion Dot : Subsystem
  qdot : Outport
  wires:
  ω/1 -> Quaternion Dot/1(ω)
  Integrating/1(Q) -> Quaternion Dot/2(q), qdot/1
  Quaternion Dot/1(Q dot) -> Integrating/1(Qdot)

== system drone_estimator_angle_dynamics/Quadrotor Dynamics/Dynamics/Quaternion Dynamics/Rotational Dynamics ==
  note: $\dot R = - \left[\omega\right]_x R$
  w : Inport
  Initial Euler Angles : Constant  Value=EulerInitialValues
  Integrator : Integrator  InitialConditionSource=external  InitialCondition=eye(3)
  Matrix Multiply1 : Product  Multiplication=Matrix(*)
  Rotation Angles to Direction Cosine Matrix : sharedtransform/Rotation Angles to Direction Cosine Matrix  rotationOrder=ZYX  aMode=aMode
  Scope : Scope
  Selector : Selector  InputPortWidth=3  IndexOptions=Index vector (dialog)  Indices=[3 2 1]  OutputSizes=1
  Skew (w) : Subsystem
  Unary Minus : UnaryMinus
  Rbe : Outport
  wires:
  Skew (w)/1(Wx) -> Unary Minus/1
  Integrator/1 -> Matrix Multiply1/2, Scope/1, Rbe/1
  Unary Minus/1 -> Matrix Multiply1/1
  Matrix Multiply1/1 -> Integrator/1
  w/1 -> Skew (w)/1(w)
  Initial Euler Angles/1 -> Selector/1
  Selector/1 -> Rotation Angles to Direction Cosine Matrix/1
  Rotation Angles to Direction Cosine Matrix/1 -> Integrator/2

== system drone_estimator_angle_dynamics/Quaternion Command/Rotation Interpolation/alpha/Guassian (a)1 ==
  In1 : Inport
  Constant1 : Constant  Value=-1/4
  Constant3 : Constant  Value=0.1
  Exp7 : Math
  Exp8 : Math  Operator=square
  Gain1 : Gain  Gain=0.9
  Product3 : Product
  Sum1 : Sum
  Out1 : Outport
  wires:
  Exp7/1 -> Gain1/1
  Constant1/1 -> Product3/2
  Constant3/1 -> Sum1/2
  Product3/1 -> Exp7/1
  In1/1 -> Exp8/1
  Sum1/1 -> Out1/1
  Gain1/1 -> Sum1/1
  Exp8/1 -> Product3/1

== system drone_estimator_angle_dynamics/Quaternion Command/Rotation Interpolation/alpha/Guassian (a)2 ==
  In1 : Inport
  Constant1 : Constant  Value=-1/4
  Constant3 : Constant  Value=0.1
  Exp7 : Math
  Exp8 : Math  Operator=square
  Gain1 : Gain  Gain=0.9
  Product3 : Product
  Sum1 : Sum
  Out1 : Outport
  wires:
  Exp8/1 -> Product3/1
  Gain1/1 -> Sum1/1
  Sum1/1 -> Out1/1
  In1/1 -> Exp8/1
  Product3/1 -> Exp7/1
  Constant3/1 -> Sum1/2
  Constant1/1 -> Product3/2
  Exp7/1 -> Gain1/1

== system drone_estimator_angle_dynamics/Quaternion Command/Rotation Interpolation/alpha/Guassian (a)3 ==
  In1 : Inport
  Constant1 : Constant  Value=-1/4
  Constant3 : Constant  Value=0.1
  Exp7 : Math
  Exp8 : Math  Operator=square
  Gain1 : Gain  Gain=0.9
  Product3 : Product
  Sum1 : Sum
  Out1 : Outport
  wires:
  Exp7/1 -> Gain1/1
  Constant1/1 -> Product3/2
  Constant3/1 -> Sum1/2
  Product3/1 -> Exp7/1
  In1/1 -> Exp8/1
  Sum1/1 -> Out1/1
  Gain1/1 -> Sum1/1
  Exp8/1 -> Product3/1

== system drone_estimator_angle_dynamics/Quadrotor Dynamics/Dynamics/Quaternion Dynamics/Quaternion Dynamics/Integrating ==
  Qdot : Inport
  Bus Creator1 : BusCreator  Inputs=q0,vec  OutDataTypeStr=Bus: QuaturnionBus
  Demux2 : Demux
  Initial Euler Angles : Constant  Value=EulerInitialValues
  Mux : Mux  Inputs=3
  Quaternion Integration : Integrator  InitialConditionSource=external  InitialCondition=[e0_0 e1_0 e2_0 e3_0]  ContinuousStateAttributes={'q0', 'q1', 'q2', 'q3'}
  Quaternion Normalize : sharedutil/Quaternion Normalize  aMode=aMode
  Rotation Angles to Quaternions : sharedtransform/Rotation Angles to Quaternions  rotationOrder=ZYX  aMode=aMode
  Selector : Selector  InputPortWidth=3  IndexOptions=Index vector (dialog)  Indices=[3 2 1]  OutputSizes=1
  Q : Outport  OutDataTypeStr=double  VectorParamsAs1DForOutWhenUnconnected=off
  wires:
  Initial Euler Angles/1 -> Selector/1
  Rotation Angles to Quaternions/1 -> Quaternion Integration/2
  Selector/1 -> Rotation Angles to Quaternions/1
  Qdot/1 -> Quaternion Integration/1
  Quaternion Integration/1 -> Quaternion Normalize/1
  Demux2/2 -> Mux/1
  Demux2/4 -> Mux/3
  Bus Creator1/1 -> Q/1
  Demux2/3 -> Mux/2
  Mux/1 -> Bus Creator1/2  "vec"
  Demux2/1 -> Bus Creator1/1  "q0"
  Quaternion Normalize/1 -> Demux2/1

== system drone_estimator_angle_dynamics/Quadrotor Dynamics/Dynamics/Quaternion Dynamics/Quaternion Dynamics/Quaternion Dot ==
  note: $\dot q_0 = -0.5 \cdot\left(w^T \cdot qvec\right) \\ \dot q_{vec} = 0.5 \cdot \left(q_0 \cdot w + q_{vec} \times w\right)$
  ω : Inport  OutDataTypeStr=double
  q : Inport  Port=2
  3x3 Cross Product : sharedutil/3x3 Cross Product  aMode=aMode
  Add : Sum  Inputs=|++
  Bus Selector1 : BusSelector  OutputSignals=q0
  Bus Selector2 : BusSelector  OutputSignals=vec
  Gain : Gain  Gain=-0.5
  Gain1 : Gain  Gain=0.5
  Mux : Mux  Inputs=2
  Product : Product
  Product1 : Product  Inputs=**  Multiplication=Matrix(*)  SaturateOnIntegerOverflow=on  OutDataTypeStr=Inherit: Same as first input
  Reshape2 : Reshape  OutputDimensionality=Column vector (2-D)
  Reshape3 : Reshape  OutputDimensionality=Row vector (2-D)
  To1D : Reshape
  To1D1 : Reshape
  Q dot : Outport
  wires:
  3x3 Cross Product/1 -> Add/1  "qvec x ω"
  Product/1 -> Add/2  "q0 * ω"
  Gain1/1 -> Mux/2
  ω/1 -> To1D1/1, Product/2, Reshape3/1
  q/1 -> Bus Selector1/1, Bus Selector2/1
  To1D1/1 -> 3x3 Cross Product/2
  To1D/1 -> 3x3 Cross Product/1
  Bus Selector2/1 -> Reshape2/1, To1D/1  "<vec>"
  Product1/1 -> Gain/1  "ω * qvec"
  Gain/1 -> Mux/1
  Bus Selector1/1 -> Product/1  "<q0>"
  Mux/1 -> Q dot/1
  Reshape2/1 -> Product1/2
  Reshape3/1 -> Product1/1
  Add/1 -> Gain1/1

== system drone_estimator_angle_dynamics/Quadrotor Dynamics/Dynamics/Quaternion Dynamics/Rotational Dynamics/Skew (w) ==
  note: $\left[\matrix{0 & -z & y \cr z & 0 & -x \cr -y & x & 0}\right]$
  w : Inport
  Constant1 : Constant  Value=0
  Constant2 : Constant  Value=0
  Constant3 : Constant  Value=0
  Demux : Demux  Outputs=3
  Matrix Concatenate : Concatenate  NumInputs=3  Mode=Multidimensional array  ConcatenateDimension=2
  Mux : Mux  Inputs=3
  Mux1 : Mux  Inputs=3
  Mux2 : Mux  Inputs=3
  Selector : Selector  InputPortWidth=3  IndexOptions=Index vector (dialog)  Indices=[3 2 1]  OutputSizes=1
  Unary Minus : UnaryMinus
  Unary Minus1 : UnaryMinus
  Unary Minus2 : UnaryMinus
  Wx : Outport
  wires:
  Constant2/1 -> Mux2/3  "0"
  Demux/1 -> Unary Minus/1, Mux/2  "z"
  Unary Minus/1 -> Mux1/1  "-z"
  Constant3/1 -> Mux/1  "0"
  Demux/3 -> Unary Minus2/1, Mux1/3  "x"
  Demux/2 -> Mux2/1, Unary Minus1/1  "y"
  Unary Minus2/1 -> Mux2/2  "-x"
  Constant1/1 -> Mux1/2  "0"
  Mux1/1 -> Matrix Concatenate/2  "c2"
  Mux/1 -> Matrix Concatenate/1  "c1"
  Mux2/1 -> Matrix Concatenate/3  "c3"
  Unary Minus1/1 -> Mux/3  "-y"
  Matrix Concatenate/1 -> Wx/1
  Selector/1 -> Demux/1
  w/1 -> Selector/1

== matlab function drone_estimator_angle_dynamics/Estimator1/Inertia Estimation/MATLAB Function ==
  data: est_dot output size=[3 3]; est input size=[3 3]; e input size=[3 1]; v input size=[3 1]; est_max input size=[3 3]; est_min input size=[3 3]; eps input
function est_dot = fcn(est, e, v, est_max, est_min, eps)
est_dot_tmp = - v * e'- e * v';
est_dot = zeros(size(est));

if norm(e) > eps
    for i = 1:length(est(:))
        est_dot(i) = EstDot(est_dot_tmp(i), est(i), est_max(i), est_min(i));
    end
end

function est_dot = EstDot(tmp, est, est_max, est_min)
    est_dot = 0;
    if (est < est_max && est > est_min) || ...
      (est > est_min && tmp < 0) || ...
      (est < est_max && tmp > 0) 
        est_dot = tmp;
    end 
end

end

== matlab function drone_estimator_angle_dynamics/Rotational Matrix Controller/Rotational Controller/MATLAB Function ==
  data: sr output size=[3 1]; wc output size=[3 1]; Kr input size=[3 3]; R input size=[3 3]; Rd input size=[3 3]; Rd_dot input size=[3 3]; Re output
function [sr, wc, Re] = fcn(Kr, R, Rd, Rd_dot)

% R_y = RotZ(Euler(3));
% R_rp = R_y * R;
% [sr_rp, wc_rp, Re_rp] = Control(R_rp, Rd, Rd_dot, Kr);

[sr, wc, Re] = Control(R, Rd, Rd_dot, Kr);

function mat = Skew(vec)
    mat = [0, -vec(3), vec(2); vec(3), 0, -vec(1); -vec(2), vec(1), 0];
end

function R = RotZ(ang)
    R = [cos(ang), -sin(ang), 0; sin(ang), cos(ang), 0; 0, 0, 1];
end

function [sr, wc, Re] = Control(R, Rd, Rd_dot, Kr)
    Re = Rd * R';
    sr = InvSkew(Re - eye(3));
    
    RdR = Rd_dot * R';
    W1 = RdR;
    W2 = Re;
    q = Skew(Kr * sr);
    
    wc = InvSkew(W2' * (-W1 - q));
end

function vec = InvSkew(mat)
    vec = zeros(3, 1);
    vec(1) = (mat(3,2) - mat(2,3)) / 2;
    vec(2) = (mat(1,3) - mat(3,1)) / 2;
    vec(3) = (mat(2,1) - mat(1,2)) / 2;
end
end

== matlab function drone_estimator_angle_dynamics/Estimator/Inertia Estimation/MATLAB Function ==
  data: est_dot output size=[3 3]; est input size=[3 3]; e input size=[3 1]; v input size=[3 1]; est_max input size=[3 3]; est_min input size=[3 3]; eps input
function est_dot = fcn(est, e, v, est_max, est_min, eps)
est_dot_tmp = - v * e'- e * v';
est_dot = zeros(size(est));

if norm(e) > eps
    for i = 1:length(est(:))
        est_dot(i) = EstDot(est_dot_tmp(i), est(i), est_max(i), est_min(i));
    end
end

function est_dot = EstDot(tmp, est, est_max, est_min)
    est_dot = 0;
    if (est < est_max && est > est_min) || ...
      (est > est_min && tmp < 0) || ...
      (est < est_max && tmp > 0) 
        est_dot = tmp;
    end 
end

end

== matlab function drone_estimator_angle_dynamics/Control Barrier Functions/CBF ==
  data: udes input size=[3 1]; fest input size=[3 1]; inertia_est input size=[3 3]; usat output size=[3 1]; w input size=[3 1]; w_min input size=1; w_max input size=1; u_min input size=1; u_max input size=1
function usat  = fcn(udes, fest, inertia_est, w, w_min, w_max, u_min, u_max)
% h1 = (xmax - x) >= 0 
%h1dot = -xdot >= - alpha (xmax - x) => u <= alpha (xmax - x)
% h2 = (x- xmin) >= 0 
%h2dot = xdot >= - alpha (x - xmin) => - u <= alpha (x - xmin)
% J = (u-udes)^2 -> J = u^2 - 2*udes*u + udes^2 
% J = 1/2 x' * H * x + f' x;
% A*x <= b
%We have two conditions:
%   u <= alpha (xmax-x)
% -u <= alpha (x - xmin)
% 
% H = [ 2 * eye(3)]; 
% f = [-2 * udes];
% theta = inv(inertia_est);
% A = [ theta;
%      -theta;
%       eye(3);
%      -eye(3)];
% alpha = 10; 
% F = fest;%0.5 * x^2;
% b = [- F + alpha*(w_max-w); 
%      + F + alpha*(w-w_min);
%       u_max*eye(3,1);
%      -u_min*eye(3,1)];
% options = optimoptions('quadprog','Algorithm','active-set');
% [u_opt] =  quadprog(H, f, A, b, [], [], [], [], udes, options);

usat = udes;
for i = 1:3
H = [ 2 * 1]; 
f = [-2 * udes(i)];
theta = inv(inertia_est);
A = [ theta(i,i);
     -theta(i,i);
      1;
     -1];
A = [1;
     -1];
alpha = 10; 
F = fest;%0.5 * x^2;
b = [- F(i) + alpha*(w_max - w(i)); 
     + F(i) + alpha*(w(i) - w_min);
      u_max;
     -u_min];
b = [u_max;
     -u_min];
options = optimoptions('quadprog','Algorithm','active-set');
[u_opt] =  quadprog(H, f, A, b, [], [], [], [], udes(i), options);
usat(i) = u_opt;
end



% if(exitflag == 1)
    % u = u_opt;
% else
    % u = 0;
% end

== matlab function drone_estimator_angle_dynamics/Rotational Matrix Controller/Rotational Controller/MATLAB Function1 ==
  data: sr output size=[3 1]; wc output size=[3 1]; Kr input size=[3 3]; R input size=[3 3]; Rd input size=[3 3]; Rd_dot input size=[3 3]; Re output
function [sr, wc, Re] = fcn(Kr, R, Rd, Rd_dot)

Re = Rd * R';
sr = 0.5 * InvSkew(Re - Re');

RdR = Rd_dot * R';
W1 = 0.5 * InvSkew(RdR - RdR');
W2 = 0.5 * (eye(3) * trace(Re') - Re');

wc = W2 \ (-W1 - Kr * sr);

function vec = InvSkew(mat)
    vec = zeros(3, 1);
    vec(1) = (mat(3,2) - mat(2,3)) / 2;
    vec(2) = (mat(1,3) - mat(3,1)) / 2;
    vec(3) = (mat(2,1) - mat(1,2)) / 2;
end
end
